simulink model "hitsi3_model"  (R2019a)
settings: Solver=VariableStepAuto  StartTime=0.0  StopTime=10.0  RelTol=1e-3
undefined symbols (not defined in the file or in its folder): K, sysC, sysKf
settings Model: Creator=akaptano  LastModifiedBy=akaptano

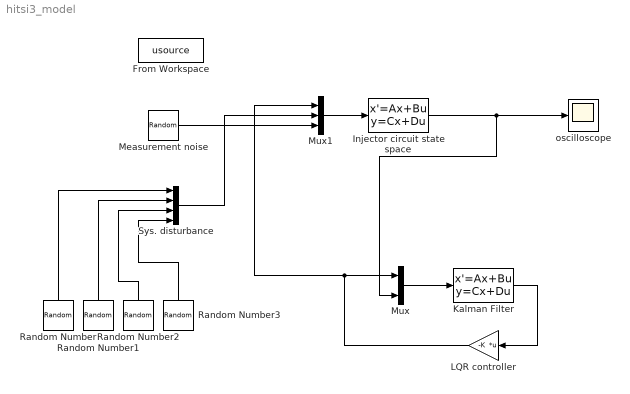
== system hitsi3_model ==
  From Workspace : FromWorkspace  VariableName=usource  SampleTime=0
  Injector circuit state space : StateSpace  A=sysC.a  B=sysC.b  C=sysC.c  D=sysC.d  InitialCondition=[0 0 0 0]
  Kalman Filter : StateSpace  A=sysKf.a  B=sysKf.b  C=sysKf.c  D=sysKf.d  InitialCondition=[0 0 0 0]
  LQR controller : Gain  Gain=-K  Multiplication=Matrix(K*u) (u vector)
  Measurement noise : RandomNumber  SampleTime=0.1
  Mux : Mux  Inputs=2
  Mux1 : Mux  Inputs=3
  Random Number{,1..3} (4 alike) : RandomNumber  SampleTime=0.1
  Sys. disturbance : Mux
  oscilloscope : Scope
  wires:
  Mux/1 -> Kalman Filter/1
  LQR controller/1 -> Mux/1, Mux1/1
  Kalman Filter/1 -> LQR controller/1
  Injector circuit state space/1 -> Mux/2, oscilloscope/1
  Mux1/1 -> Injector circuit state space/1
  Measurement noise/1 -> Mux1/3
  Random Number3/1 -> Sys. disturbance/4
  Random Number2/1 -> Sys. disturbance/3
  Random Number1/1 -> Sys. disturbance/2
  Random Number/1 -> Sys. disturbance/1
  Sys. disturbance/1 -> Mux1/2
